simulink model "GATE_C"  (R2016a)
settings: Solver=FixedStepDiscrete  StartTime=0.0  StopTime=120  RelTol=1e-3
values from neighbouring files (symbols this model uses):
  CLOSE_SIDE_VALUE = single(4*ONE_SEC)    [GateParameter.m]
  CLOSED = uint8(12)    [GateParameter.m]
  CLOSING = uint8(13)    [GateParameter.m]
  CURRENT_STABLE_TIMER = uint8(200)    [GateParameter.m]
  CURRENT_THRESH = uint16(1000)    [GateParameter.m]
  INIT = uint8(15)    [GateParameter.m]
  MOVING_TIMER = uint32(60*ONE_SEC)    [GateParameter.m]
  OPEN = uint8(14)    [GateParameter.m]
  OPEN_SIDE_VALUE = uint16(4*ONE_SEC)    [GateParameter.m]
  OPENING = uint8(11)    [GateParameter.m]
  OPENING_ACTIVE = uint8(1)    [GateParameter.m]
  STABLE_TIMER_VALUE = uint16(1*ONE_SEC)    [GateParameter.m]
settings Model: ExtModeTrigDuration=2  Creator=omaro  LastModifiedBy=oelkawok
settings DataIOCC: SaveFormat=StructureWithTime  SaveOutput=off  SaveTime=off
settings OptimizationCC: DefaultParameterBehavior=Inlined  StateBitsets=on  DataBitsets=on  LifeSpan=1  MaxStackSize=64
settings DebuggingCC: ConsistencyChecking=error  SignalInfNanChecking=error  SignalRangeChecking=error  ReadBeforeWriteMsg=EnableAllAsError  WriteAfterWriteMsg=EnableAllAsError  WriteAfterReadMsg=EnableAllAsError  AlgebraicLoopMsg=error  ArtificialAlgebraicLoopMsg=error  BlockPriorityViolationMsg=error  MinStepSizeMsg=error  CheckMatrixSingularityMsg=error  ParameterUnderflowMsg=error  ParameterPrecisionLossMsg=error  UnderSpecifiedDataTypeMsg=warning  UnnecessaryDatatypeConvMsg=warning  VectorMatrixConversionMsg=error  SignalLabelMismatchMsg=error  UnconnectedInputMsg=error  UnconnectedOutputMsg=error  UnconnectedLineMsg=error  SFcnCompatibilityMsg=error  UniqueDataStoreMsg=error  BusObjectLabelMismatch=error  RootOutportRequireBusObject=error  ModelReferenceIOMsg=error  ModelReferenceVersionMismatchMessage=error  ModelReferenceIOMismatchMessage=error  ModelReferenceDataLoggingMessage=error  StrictBusMsg=ErrorOnBusTreatedAsVector  SFUnusedDataAndEventsDiag=error  SFUnexpectedBacktrackingDiag=error  SFInvalidInputDataAccessInChartInitDiag=error  SFNoUnconditionalDefaultTransitionDiag=error  SFTransitionOutsideNaturalParentDiag=error  SFUndirectedBroadcastEventsDiag=error  SFTransitionActionBeforeConditionDiag=error  SFOutputUsedAsStateInMooreChartDiag=warning
settings HardwareCC: ProdBitPerInt=16  ProdBitPerPointer=16  ProdLargestAtomicFloat=None  ProdWordSize=8  ProdHWDeviceType=Atmel->AVR
settings SFSimCC: SimCustomHeaderCode=|
  | //#include "C:\Users\omaro\Desktop\Gate_Model\Arduino\Arduino.h"
  | //#include "Keypad\Keypad.h"
settings RTWCC: SystemTargetFile=ert.tlc  TemplateMakefile=ert_default_tmf  GenerateReport=on  RTWUseSimCustomCode=on  Toolchain=Arduino AVR v1.6.1  BuildConfiguration=Faster Runs  LaunchReport=on
settings RTWCC: CustomHeaderCode=|
  | //#include "C:\Users\omaro\Desktop\Gate_Model\Arduino\Arduino.h"
  | //#include "Keypad\Keypad.h"
settings CodeAppCC: ForceParamTrailComments=on  OperatorAnnotations=on  MATLABSourceComments=on
settings ERTTargetCC: ERTCustomFileBanners=off  SupportContinuousTime=on  SupportNonInlinedSFcns=on  SupportVariableSizeSignals=on  ModelStepFunctionPrototypeControlCompliant=off  RootIOFormat=Structure reference  ERTCustomFileTemplate=example_file_process.tlc

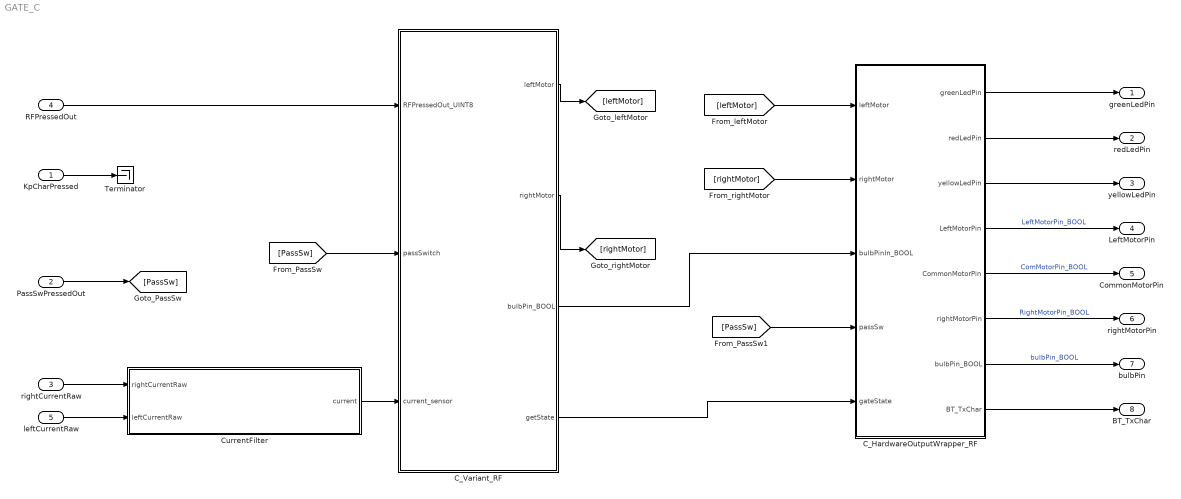
== system GATE_C ==
  KpCharPressed : Inport  OutDataTypeStr=uint8  PortDimensions=1  SampleTime=0
  PassSwPressedOut : Inport  Port=2  OutDataTypeStr=boolean  PortDimensions=1  SampleTime=0
  rightCurrentRaw : Inport  Port=3  OutDataTypeStr=uint16  PortDimensions=1  SampleTime=0
  RFPressedOut : Inport  Port=4  OutDataTypeStr=uint8  PortDimensions=1  SampleTime=0
  leftCurrentRaw : Inport  Port=5  OutDataTypeStr=uint16  PortDimensions=1  SampleTime=0
  C_HardwareOutputWrapper_RF : Subsystem  VariantControl=Variant3
  C_Variant_RF : Subsystem  VariantControl=Variant3
  CurrentFilter : Subsystem
  Terminator : Terminator
  greenLedPin : Outport  OutDataTypeStr=double  PortDimensions=1  SampleTime=[0.001,0]
  redLedPin : Outport  Port=2  OutDataTypeStr=double  PortDimensions=1  SampleTime=[0.001,0]
  yellowLedPin : Outport  Port=3  OutDataTypeStr=double  PortDimensions=1  SampleTime=[0.001,0]
  LeftMotorPin : Outport  Port=4  OutDataTypeStr=boolean  PortDimensions=1  SampleTime=[0.001,0]
  CommonMotorPin : Outport  Port=5  OutDataTypeStr=boolean  PortDimensions=1  SampleTime=[0.001,0]
  rightMotorPin : Outport  Port=6  OutDataTypeStr=boolean  PortDimensions=1  SampleTime=[0.001,0]
  bulbPin : Outport  Port=7  OutDataTypeStr=boolean  PortDimensions=1  SampleTime=[0.001,0]
  BT_TxChar : Outport  Port=8  OutDataTypeStr=double  PortDimensions=1  SampleTime=[0.001,0]
  wires:
  PassSwPressedOut/1 -> [PassSw]
  KpCharPressed/1 -> Terminator/1
  [PassSw] -> C_Variant_RF/2(passSwitch)
  rightCurrentRaw/1 -> CurrentFilter/1(rightCurrentRaw)
  C_Variant_RF/1(leftMotor) -> [leftMotor]
  C_Variant_RF/2(rightMotor) -> [rightMotor]
  [leftMotor] -> C_HardwareOutputWrapper_RF/1(leftMotor)
  [rightMotor] -> C_HardwareOutputWrapper_RF/2(rightMotor)
  C_Variant_RF/3(bulbPin_BOOL) -> C_HardwareOutputWrapper_RF/3(bulbPinIn_BOOL)
  [PassSw] -> C_HardwareOutputWrapper_RF/4(passSw)
  C_HardwareOutputWrapper_RF/1(greenLedPin) -> greenLedPin/1
  C_HardwareOutputWrapper_RF/2(redLedPin) -> redLedPin/1
  C_HardwareOutputWrapper_RF/3(yellowLedPin) -> yellowLedPin/1
  C_HardwareOutputWrapper_RF/4(LeftMotorPin) -> LeftMotorPin/1  "LeftMotorPin_BOOL"
  C_HardwareOutputWrapper_RF/5(CommonMotorPin) -> CommonMotorPin/1  "ComMotorPin_BOOL"
  C_HardwareOutputWrapper_RF/6(rightMotorPin) -> rightMotorPin/1  "RightMotorPin_BOOL"
  C_HardwareOutputWrapper_RF/7(bulbPin_BOOL) -> bulbPin/1  "bulbPin_BOOL"
  C_HardwareOutputWrapper_RF/8(BT_TxChar) -> BT_TxChar/1
  CurrentFilter/1(current) -> C_Variant_RF/3(current_sensor)
  leftCurrentRaw/1 -> CurrentFilter/2(leftCurrentRaw)
  RFPressedOut/1 -> C_Variant_RF/1(RFPressedOut_UINT8)
  C_Variant_RF/4(getState) -> C_HardwareOutputWrapper_RF/5(gateState)

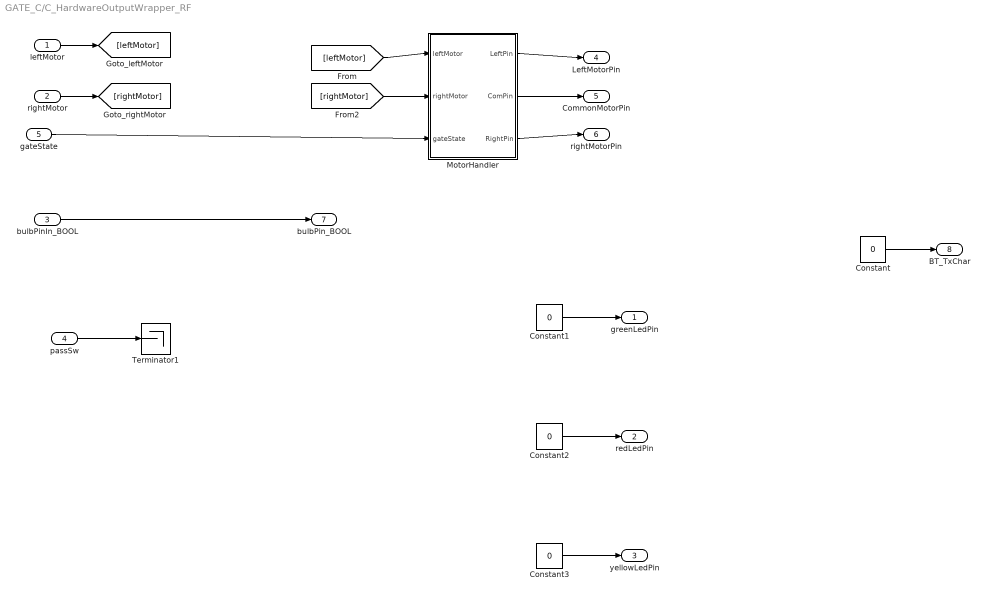
== system GATE_C/C_HardwareOutputWrapper_RF ==
  leftMotor : Inport
  rightMotor : Inport  Port=2
  bulbPinIn_BOOL : Inport  Port=3
  passSw : Inport  Port=4
  gateState : Inport  Port=5
  Constant{,1..3} (4 alike) : Constant  Value=0  SampleTime=-1
  MotorHandler : Subsystem
  Terminator1 : Terminator
  greenLedPin : Outport
  redLedPin : Outport  Port=2
  yellowLedPin : Outport  Port=3
  LeftMotorPin : Outport  Port=4
  CommonMotorPin : Outport  Port=5
  rightMotorPin : Outport  Port=6
  bulbPin_BOOL : Outport  Port=7
  BT_TxChar : Outport  Port=8
  wires:
  passSw/1 -> Terminator1/1
  Constant1/1 -> greenLedPin/1
  Constant2/1 -> redLedPin/1
  Constant3/1 -> yellowLedPin/1
  Constant/1 -> BT_TxChar/1
  rightMotor/1 -> [rightMotor]
  leftMotor/1 -> [leftMotor]
  bulbPinIn_BOOL/1 -> bulbPin_BOOL/1
  MotorHandler/3(RightPin) -> rightMotorPin/1
  MotorHandler/2(ComPin) -> CommonMotorPin/1
  MotorHandler/1(LeftPin) -> LeftMotorPin/1
  [rightMotor] -> MotorHandler/2(rightMotor)
  [leftMotor] -> MotorHandler/1(leftMotor)
  gateState/1 -> MotorHandler/3(gateState)

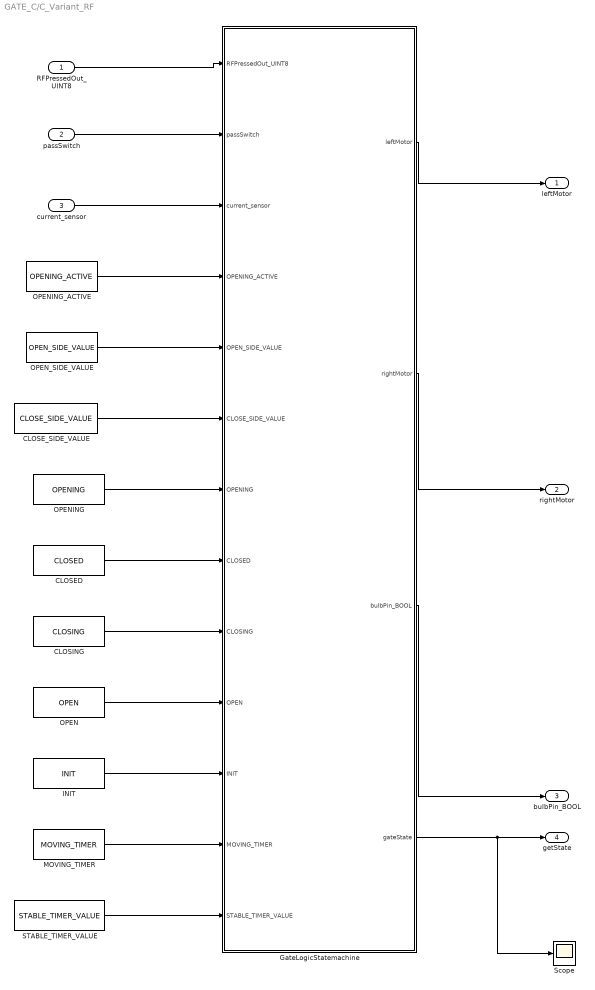
== system GATE_C/C_Variant_RF ==
  RFPressedOut_UINT8 : Inport
  passSwitch : Inport  Port=2
  current_sensor : Inport  Port=3
  CLOSED : Constant  Value=CLOSED  SampleTime=-1
  CLOSE_SIDE_VALUE : Constant  Value=CLOSE_SIDE_VALUE  SampleTime=-1
  CLOSING : Constant  Value=CLOSING  SampleTime=-1
  GateLogicStatemachine : Stateflow chart  TreatAsAtomicUnit=on
  INIT : Constant  Value=INIT  SampleTime=-1
  MOVING_TIMER : Constant  Value=MOVING_TIMER  SampleTime=-1
  OPEN : Constant  Value=OPEN  SampleTime=-1
  OPENING : Constant  Value=OPENING  SampleTime=-1
  OPENING_ACTIVE : Constant  Value=OPENING_ACTIVE  SampleTime=-1
  OPEN_SIDE_VALUE : Constant  Value=OPEN_SIDE_VALUE  SampleTime=-1
  STABLE_TIMER_VALUE : Constant  Value=STABLE_TIMER_VALUE  SampleTime=-1
  Scope : Scope
  leftMotor : Outport
  rightMotor : Outport  Port=2
  bulbPin_BOOL : Outport  Port=3
  getState : Outport  Port=4
  wires:
  CLOSING/1 -> GateLogicStatemachine/9(CLOSING)
  OPENING/1 -> GateLogicStatemachine/7(OPENING)
  CLOSED/1 -> GateLogicStatemachine/8(CLOSED)
  OPEN/1 -> GateLogicStatemachine/10(OPEN)
  RFPressedOut_UINT8/1 -> GateLogicStatemachine/1(RFPressedOut_UINT8)
  GateLogicStatemachine/3(bulbPin_BOOL) -> bulbPin_BOOL/1
  current_sensor/1 -> GateLogicStatemachine/3(current_sensor)
  GateLogicStatemachine/1(leftMotor) -> leftMotor/1
  GateLogicStatemachine/2(rightMotor) -> rightMotor/1
  OPENING_ACTIVE/1 -> GateLogicStatemachine/4(OPENING_ACTIVE)
  OPEN_SIDE_VALUE/1 -> GateLogicStatemachine/5(OPEN_SIDE_VALUE)
  CLOSE_SIDE_VALUE/1 -> GateLogicStatemachine/6(CLOSE_SIDE_VALUE)
  passSwitch/1 -> GateLogicStatemachine/2(passSwitch)
  INIT/1 -> GateLogicStatemachine/11(INIT)
  MOVING_TIMER/1 -> GateLogicStatemachine/12(MOVING_TIMER)
  STABLE_TIMER_VALUE/1 -> GateLogicStatemachine/13(STABLE_TIMER_VALUE)
  GateLogicStatemachine/4(gateState) -> Scope/1, getState/1

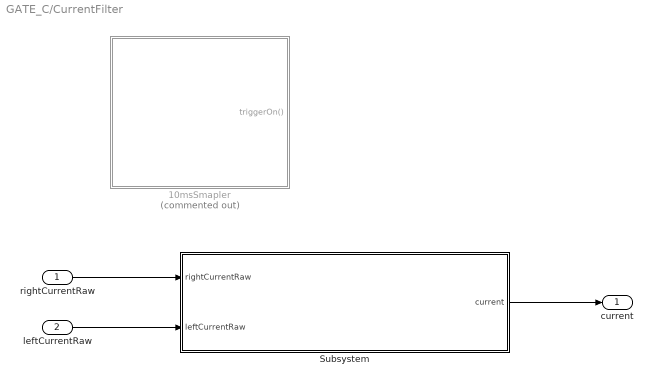
== system GATE_C/CurrentFilter ==
  rightCurrentRaw : Inport
  leftCurrentRaw : Inport  Port=2
  10msSmapler : Stateflow chart  Commented=on  TreatAsAtomicUnit=on
  Subsystem : Subsystem
  current : Outport
  wires:
  leftCurrentRaw/1 -> Subsystem/2(leftCurrentRaw)
  rightCurrentRaw/1 -> Subsystem/1(rightCurrentRaw)
  Subsystem/1(current) -> current/1

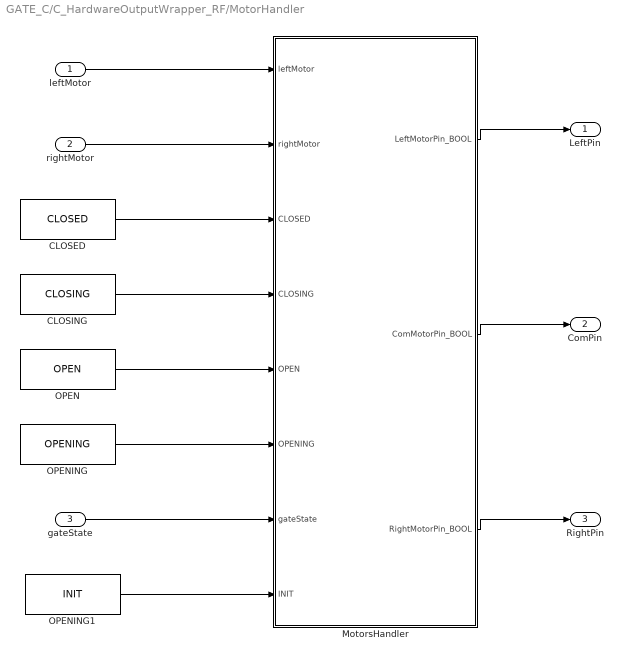
== system GATE_C/C_HardwareOutputWrapper_RF/MotorHandler ==
  leftMotor : Inport
  rightMotor : Inport  Port=2
  gateState : Inport  Port=3
  CLOSED : Constant  Value=CLOSED  SampleTime=-1
  CLOSING : Constant  Value=CLOSING  SampleTime=-1
  MotorsHandler : Stateflow chart  TreatAsAtomicUnit=on
  OPEN : Constant  Value=OPEN  SampleTime=-1
  OPENING : Constant  Value=OPENING  SampleTime=-1
  OPENING1 : Constant  Value=INIT  SampleTime=-1
  LeftPin : Outport
  ComPin : Outport  Port=2
  RightPin : Outport  Port=3
  wires:
  OPENING1/1 -> MotorsHandler/8(INIT)
  leftMotor/1 -> MotorsHandler/1(leftMotor)
  gateState/1 -> MotorsHandler/7(gateState)
  MotorsHandler/3(RightMotorPin_BOOL) -> RightPin/1
  MotorsHandler/2(ComMotorPin_BOOL) -> ComPin/1
  MotorsHandler/1(LeftMotorPin_BOOL) -> LeftPin/1
  OPENING/1 -> MotorsHandler/6(OPENING)
  OPEN/1 -> MotorsHandler/5(OPEN)
  CLOSING/1 -> MotorsHandler/4(CLOSING)
  CLOSED/1 -> MotorsHandler/3(CLOSED)
  rightMotor/1 -> MotorsHandler/2(rightMotor)

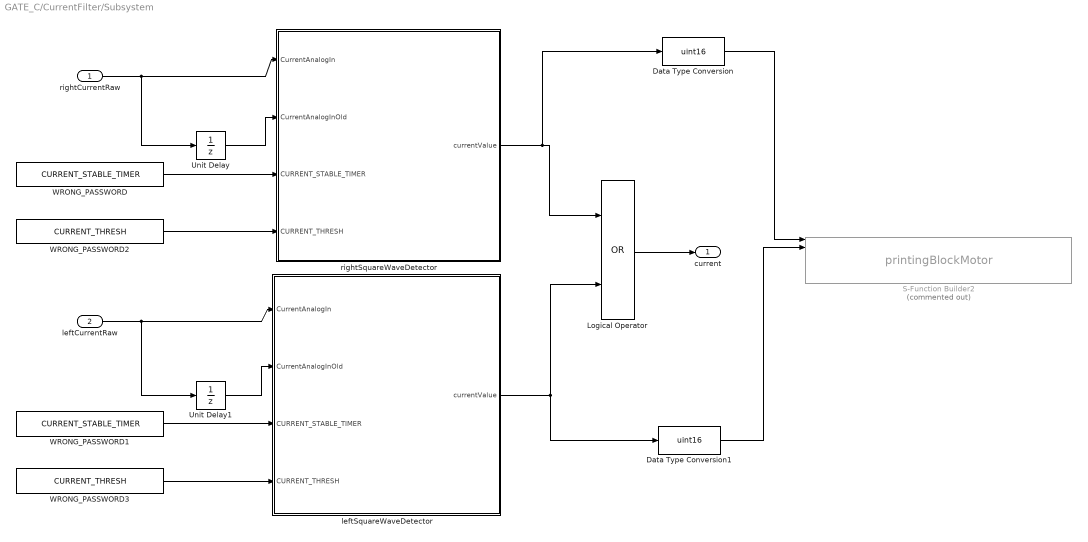
== system GATE_C/CurrentFilter/Subsystem ==
  rightCurrentRaw : Inport
  leftCurrentRaw : Inport  Port=2
  Data Type Conversion : DataTypeConversion  OutDataTypeStr=uint16
  Data Type Conversion1 : DataTypeConversion  OutDataTypeStr=uint16
  Logical Operator : Logic  Operator=OR  AllPortsSameDT=off  OutDataTypeStr=boolean
  S-Function Builder2 : S-Function  Commented=on  InitFcn=try, set_param(gcb,'FunctionName','printingBlockMotor'), end  FunctionName=printingBlockMotor  SFunctionModules=printingBlockMotor_wrapper  SFunctionDeploymentMode=off  EnableBusSupport=off  mask(S-Function Builder){}
      mask help: Simulink:masks:SFunctionBuilder_MD
      mask init:
      | val = [[.9  0.75 0.75 1 1 .9 .9 1]',[1 1 0.75 0.75 .9 .9 1 .9]'];try , sys = get_param(gcb,'SfunBuilderFcnName');if isempty(sys), sys = get_param(gcb,'FunctionName'); end,catch, sys = get_param(gcb,'FunctionName'); end
      settings: CopyFcn=set_param(gcbh,'LinkStatus','none')  PreSaveFcn=try, set_param(gcb,'FunctionName','printingBlockMotor'), end  OpenFcn=sfunctionwizard(gcbh)
      mask Display: plot(val(:,1),val(:,2)),disp(sys), port_label('input',1,'u0'), port_label('input',2,'u1')
  Unit Delay : UnitDelay  SampleTime=-1
  Unit Delay1 : UnitDelay  SampleTime=-1
  WRONG_PASSWORD : Constant  Value=CURRENT_STABLE_TIMER  SampleTime=-1
  WRONG_PASSWORD1 : Constant  Value=CURRENT_STABLE_TIMER  SampleTime=-1
  WRONG_PASSWORD2 : Constant  Value=CURRENT_THRESH  SampleTime=-1
  WRONG_PASSWORD3 : Constant  Value=CURRENT_THRESH  SampleTime=-1
  leftSquareWaveDetector : Stateflow chart  TreatAsAtomicUnit=on
  rightSquareWaveDetector : Stateflow chart  TreatAsAtomicUnit=on
  current : Outport
  wires:
  WRONG_PASSWORD3/1 -> leftSquareWaveDetector/4(CURRENT_THRESH)
  WRONG_PASSWORD2/1 -> rightSquareWaveDetector/4(CURRENT_THRESH)
  WRONG_PASSWORD1/1 -> leftSquareWaveDetector/3(CURRENT_STABLE_TIMER)
  WRONG_PASSWORD/1 -> rightSquareWaveDetector/3(CURRENT_STABLE_TIMER)
  Data Type Conversion1/1 -> S-Function Builder2/2
  Data Type Conversion/1 -> S-Function Builder2/1
  Logical Operator/1 -> current/1
  leftSquareWaveDetector/1(currentValue) -> Data Type Conversion1/1, Logical Operator/2
  rightSquareWaveDetector/1(currentValue) -> Logical Operator/1, Data Type Conversion/1
  Unit Delay1/1 -> leftSquareWaveDetector/2(CurrentAnalogInOld)
  leftCurrentRaw/1 -> leftSquareWaveDetector/1(CurrentAnalogIn), Unit Delay1/1
  Unit Delay/1 -> rightSquareWaveDetector/2(CurrentAnalogInOld)
  rightCurrentRaw/1 -> Unit Delay/1, rightSquareWaveDetector/1(CurrentAnalogIn)

== stateflow chart GATE_C/CurrentFilter/Subsystem/leftSquareWaveDetector ==
  state Running
    entry:
    counterHigh = 0;
    counterLow= 0;
    currentValue = 1;
    state High
      entry:
      counterLow = 0;
    state Low
      entry:
      counterHigh = 0;
    (default) -> High
    High -> High [order 2] : [CurrentAnalogIn > CURRENT_THRESH]
        | /counterHigh++;
    High -> Low [order 1] : [CurrentAnalogIn < CURRENT_THRESH]
    Low -> High [order 1] : [CurrentAnalogIn > CURRENT_THRESH]
    Low -> Low [order 2] : [CurrentAnalogIn < CURRENT_THRESH]
        | /counterLow++;
  state Stop
    entry:
    currentValue = 0;
    stableCounter = 0;
  (default) -> Stop
  Stop -> Running : [((CurrentAnalogInOld > CURRENT_THRESH)...
      |  && (CurrentAnalogIn < CURRENT_THRESH)) ...
      | || ((CurrentAnalogInOld < CURRENT_THRESH)...
      |  && (CurrentAnalogIn > CURRENT_THRESH))]
  Running -> Stop : [(counterHigh >= CURRENT_STABLE_TIMER)...
      |  || (counterLow >= CURRENT_STABLE_TIMER)]
  data: CurrentAnalogIn input; currentValue output uint8; counterHigh local uint16; counterLow local uint16; stableCounter local uint8; CurrentAnalogInOld input; CURRENT_STABLE_TIMER input; CURRENT_THRESH input

== stateflow chart GATE_C/C_HardwareOutputWrapper_RF/MotorHandler/MotorsHandler ==
  state MonitorChange
  state UpdatePins
    (default) -> (junction 91) : /* updating motor Pins Switch case */
    (junction 91) -> (junction 92) [order 1] : [(leftMotor == OPENING) && ((rightMotor == CLOSED) || (rightMotor == OPEN))]
    (junction 92) -> (junction 100) : {LeftMotorPin_BOOL = true;...
        | ComMotorPin_BOOL = true;...
        | RightMotorPin_BOOL = false;}
    (junction 91) -> (junction 93) [order 2]
    (junction 93) -> (junction 94) [order 1] : [(leftMotor == CLOSING) && ((rightMotor == CLOSED) || (rightMotor == OPEN))]
    (junction 94) -> (junction 99) : {LeftMotorPin_BOOL = false;...
        | ComMotorPin_BOOL = false;...
        |  RightMotorPin_BOOL = true;}
    (junction 93) -> (junction 95) [order 2]
    (junction 95) -> (junction 96) [order 1] : [(rightMotor == CLOSING) && ((leftMotor == CLOSED) || (leftMotor == OPEN))]
    (junction 96) -> (junction 98) : {LeftMotorPin_BOOL = true;...
        | ComMotorPin_BOOL = false;...
        | RightMotorPin_BOOL = false;}
    (junction 95) -> (junction 102) [order 2]
    (junction 102) -> (junction 103) [order 1] : [(rightMotor == OPENING) && ((leftMotor == CLOSED) || (leftMotor == OPEN))]
    (junction 103) -> (junction 110) : {LeftMotorPin_BOOL = false;...
        | ComMotorPin_BOOL = true;...
        | RightMotorPin_BOOL = true;}
    (junction 102) -> (junction 104) [order 2]
    (junction 104) -> (junction 105) [order 1] : [(rightMotor == OPENING) && (leftMotor == OPENING)]
    (junction 105) -> (junction 111) : {LeftMotorPin_BOOL = true;...
        | ComMotorPin_BOOL = true;...
        | RightMotorPin_BOOL = true;}
    (junction 104) -> (junction 106) [order 2]
    (junction 106) -> (junction 107) [order 1] : [(rightMotor == CLOSING) && (leftMotor == CLOSING)]
    (junction 106) -> (junction 123) [order 2]
    (junction 107) -> (junction 112) : {LeftMotorPin_BOOL = false;...
        | ComMotorPin_BOOL = false;...
        | RightMotorPin_BOOL = false;}
    (junction 123) -> (junction 124) [order 1] : [((rightMotor == CLOSED) || (rightMotor == OPEN)) ...
        | && ((leftMotor == CLOSED) || (leftMotor == OPEN))]
    (junction 123) -> (junction 136) [order 2]
    (junction 124) -> (junction 125) : {LeftMotorPin_BOOL = false;...
        | ComMotorPin_BOOL = true;...
        | RightMotorPin_BOOL = false;}
    (junction 136) -> (junction 138) [order 1] : [(gateState == CLOSED) || (gateState == OPEN) || (gateState == INIT)]
    (junction 136) -> (junction 97) [order 2]
    (junction 138) -> (junction 139) : {LeftMotorPin_BOOL = false;...
        | ComMotorPin_BOOL = true;...
        | RightMotorPin_BOOL = false;}
    (junction 100) -> (junction 99)
    (junction 99) -> (junction 98)
    (junction 98) -> (junction 110)
    (junction 139) -> (junction 97)
    (junction 125) -> (junction 139)
    (junction 112) -> (junction 125)
    (junction 111) -> (junction 112)
    (junction 110) -> (junction 111)
    (junction 97) -> (junction 101)
  (default) -> MonitorChange
  UpdatePins -> MonitorChange
  MonitorChange -> UpdatePins : [(hasChanged(leftMotor)) ...
      | || (hasChanged(rightMotor))...
      | || (hasChanged(gateState) && (gateState == CLOSED))...
      |  || (hasChanged(gateState) && (gateState == OPEN))...
      | ||(hasChanged(gateState) && (gateState == INIT))]
  data: leftMotor input; LeftMotorPin_BOOL output boolean =false; ComMotorPin_BOOL output boolean =true; RightMotorPin_BOOL output boolean =false; rightMotor input; CLOSED input; CLOSING input; OPEN input; OPENING input; gateState input; INIT input

== stateflow chart GATE_C/CurrentFilter/10msSmapler ==
  (default) -> (junction 2)
  (junction 2) -> (junction 3) : {counter_1ms++;}
  (junction 3) -> (junction 6) : [counter_1ms == 10]
      | {
      | triggerOn;
      | counter_1ms = 0;
      | }
  data: counter_1ms local double
  events: triggerOn output FUNCTION_CALL_EVENT

== stateflow chart GATE_C/CurrentFilter/Subsystem/rightSquareWaveDetector ==
  state Running
    entry:
    counterHigh = 0;
    counterLow= 0;
    currentValue = 1;
    state High
      entry:
      counterLow = 0;
    state Low
      entry:
      counterHigh = 0;
    (default) -> High
    High -> High [order 2] : [CurrentAnalogIn > CURRENT_THRESH]
        | /counterHigh++;
    High -> Low [order 1] : [CurrentAnalogIn < CURRENT_THRESH]
    Low -> High [order 1] : [CurrentAnalogIn > CURRENT_THRESH]
    Low -> Low [order 2] : [CurrentAnalogIn < CURRENT_THRESH]
        | /counterLow++;
  state Stop
    entry:
    currentValue = 0;
    stableCounter = 0;
  (default) -> Stop
  Stop -> Running : [((CurrentAnalogInOld > CURRENT_THRESH)...
      |  && (CurrentAnalogIn < CURRENT_THRESH)) ...
      | || ((CurrentAnalogInOld < CURRENT_THRESH)...
      |  && (CurrentAnalogIn > CURRENT_THRESH))]
  Running -> Stop : [(counterHigh >= CURRENT_STABLE_TIMER)...
      |  || (counterLow >= CURRENT_STABLE_TIMER)]
  data: CurrentAnalogIn input; currentValue output uint8; counterHigh local uint16; counterLow local uint16; stableCounter local uint8; CurrentAnalogInOld input; CURRENT_STABLE_TIMER input; CURRENT_THRESH input

== stateflow chart GATE_C/C_Variant_RF/GateLogicStatemachine ==
  state init
    entry:
    gotoReady = false;
    bulbPin_BOOL = 0;
    leftMotor = CLOSED;
    rightMotor = CLOSED;
    gateState = INIT;
  state opening
    entry:
    bulbPin_BOOL = true;
    gateState = OPENING;
    stableTimer = 0;
    during:
    openingTimer++;
    state openLeftSide
      entry:
      leftMotor = OPENING;
      openSideDelay = 0;
      during:
      openSideDelay++;
    state openRightSide
      entry:
      rightMotor = OPENING;
      du:
      stableTimer++;
    (default) -> openLeftSide
    openLeftSide -> openRightSide : [openSideDelay == OPEN_SIDE_VALUE]
  state closed
    entry:
    bulbPin_BOOL = false;
    leftMotor = CLOSED;
    rightMotor = CLOSED;
    openingActive = 0;
    gateState = CLOSED;
    closingTimer = 0;
    stableTimer = 0;
    state openingGate
      entry:
      openingActive = OPENING_ACTIVE;
    state MonitorInput
    (default) -> MonitorInput
    MonitorInput -> openingGate [order 1] : [hasChanged(RFPressedOut_UINT8) && (RFPressedOut_UINT8 == true)]
    MonitorInput -> openingGate [order 2] : [((passSwitch == true) && hasChanged(passSwitch))]
  state closing
    entry:
    gateState = CLOSING;
    du:
    closingTimer++;
    state closingRightSide
      entry:
      rightMotor = CLOSING;
      closeSideDelay = 0;
      during:
      closeSideDelay++;
    state closingLeftSide
      entry:
      leftMotor = CLOSING;
      du:
      stableTimer++;
    (default) -> closingRightSide
    closingRightSide -> closingLeftSide : [closeSideDelay == CLOSE_SIDE_VALUE]
  state open
    entry:
    gateState = OPEN;
    openingTimer = 0;
    stableTimer = 0;
    state gateOpen
      entry:
      closing_active = false;
      leftMotor = OPEN;
      rightMotor = OPEN;
    state closing
      entry:
      closing_active = true;
    (default) -> gateOpen
    gateOpen -> open.closing [order 2] : [((passSwitch == true) && hasChanged(passSwitch))]
    gateOpen -> open.closing [order 1] : [hasChanged(RFPressedOut_UINT8) && (RFPressedOut_UINT8 == true)]
  (default) -> init
  closed -> opening : [openingActive == OPENING_ACTIVE]
  init -> closed
  closing -> closed [order 1] : [(current_sensor == 0)...
      | &&(stableTimer >= STABLE_TIMER_VALUE)]
  closing -> closed [order 3] : [closingTimer >= MOVING_TIMER]
  closing -> closed [order 2] : [((hasChanged(RFPressedOut_UINT8)...
      | &&(RFPressedOut_UINT8 == true)) ...
      | || ((passSwitch == true)...
      |  && hasChanged(passSwitch)))...
      | && (stableTimer >= STABLE_TIMER_VALUE)]
  opening -> open [order 2] : [((hasChanged(RFPressedOut_UINT8)...
      | &&(RFPressedOut_UINT8 == true)) ...
      | || ((passSwitch == true)...
      |  && hasChanged(passSwitch)))...
      | && (stableTimer >= STABLE_TIMER_VALUE)]
  opening -> open [order 3] : [openingTimer >= MOVING_TIMER]
  opening -> open [order 1] : [(current_sensor == 0)...
      | && (stableTimer >= STABLE_TIMER_VALUE)]
  open -> closing : [closing_active == true]
  data: RFPressedOut_UINT8 input; openingActive local uint8; passSwitch input; closing_active local uint8; current_sensor input; openSideDelay local uint16; leftMotor output uint8 =0; rightMotor output uint8 =0; bulbPin_BOOL output boolean; closeSideDelay local uint16; OPENING_ACTIVE input =2; OPEN_SIDE_VALUE input =20; CLOSE_SIDE_VALUE input =20; OPENING input =2; CLOSED input =1; CLOSING input =4; OPEN input =3; gotoReady local boolean; gateState output uint8; closingTimer local uint32; openingTimer local uint32; stableTimer local uint32; INIT input; MOVING_TIMER input; STABLE_TIMER_VALUE input
